simulink model "seminar3_1"  (R2019b)
settings: Solver=VariableStepAuto  StartTime=0.0  StopTime=0.1  RelTol=1e-3  EnableMultiTasking=on
model workspace (MAT data in the model file):
  thit = 150
values from neighbouring files (symbols this model uses):
  fai = i*10    [Untitled.m]
libraries: powerlib x16, powerlib_meascontrol x7
settings Model: Creator=Double Rui  LastModifiedBy=96547
settings DataIOCC: ReturnWorkspaceOutputs=off
settings OptimizationCC: LifeSpan=inf
settings DebuggingCC: SFUnexpectedBacktrackingDiag=warning  SFNoUnconditionalDefaultTransitionDiag=warning  ArithmeticOperatorsInVariantConditions=warning
settings SFSimCC: SimUseLocalCustomCode=off  CustomCodeUndefinedFunction=UseInterfaceOnly
settings RTWCC: RTWUseLocalCustomCode=off
settings CodeAppCC: StateflowObjectComments=on
settings GRTTargetCC: TargetLangStandard=C89/C90 (ANSI)  GeneratePreprocessorConditionals=Disable all
settings ConfigComp: CovMetricSettings=dw  CovHtmlReporting=on  CovSaveCumulativeToWorkspaceVar=on  CovSaveSingleToWorkspaceVar=on  CovExternalEMLEnable=off
settings SimscapeCC: SimscapeNormalizeSystem=off

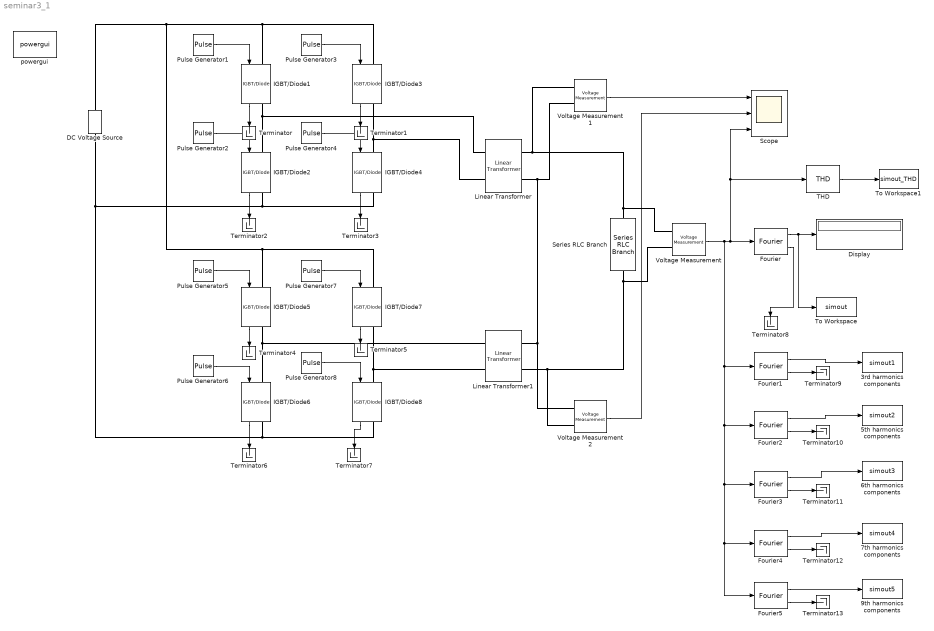
== system seminar3_1 ==
  3rd harmonics components : ToWorkspace  VariableName=simout1  SaveFormat=Timeseries  SampleTime=-1
  5th harmonics components : ToWorkspace  VariableName=simout2  SaveFormat=Timeseries  SampleTime=-1
  6th harmonics components : ToWorkspace  VariableName=simout3  SaveFormat=Timeseries  SampleTime=-1
  7th harmonics components : ToWorkspace  VariableName=simout4  SaveFormat=Timeseries  SampleTime=-1
  9th harmonics components : ToWorkspace  VariableName=simout5  SaveFormat=Timeseries  SampleTime=-1
  DC Voltage Source : powerlib/Electrical Sources/DC Voltage Source  Amplitude=400  Measurements=None
      settings: SourceProductName=Simscape Electrical
  Display : Display
  Fourier : powerlib_meascontrol/Measurements/Fourier  Freq=50  n=1  InInit=[0, 0]  Ts=0
      settings: SourceProductName=Simscape Electrical
  Fourier1 : powerlib_meascontrol/Measurements/Fourier  Freq=50  n=3  InInit=[0, 0]  Ts=0
      settings: SourceProductName=Simscape Electrical
  Fourier2 : powerlib_meascontrol/Measurements/Fourier  Freq=50  n=5  InInit=[0, 0]  Ts=0
      settings: SourceProductName=Simscape Electrical
  Fourier3 : powerlib_meascontrol/Measurements/Fourier  Freq=50  n=6  InInit=[0, 0]  Ts=0
      settings: SourceProductName=Simscape Electrical
  Fourier4 : powerlib_meascontrol/Measurements/Fourier  Freq=50  n=7  InInit=[0, 0]  Ts=0
      settings: SourceProductName=Simscape Electrical
  Fourier5 : powerlib_meascontrol/Measurements/Fourier  Freq=50  n=9  InInit=[0, 0]  Ts=0
      settings: SourceProductName=Simscape Electrical
  IGBT/Diode{1..8} (8 alike) : powerlib/Power Electronics/IGBT//Diode  Ron=1e-3  Rs=1e5  Cs=inf  Measurements=on
      settings: SourceProductName=Simscape Electrical
  Linear Transformer : powerlib/Elements/Linear Transformer  UNITS=pu  NominalPower=[ 250e6 50 ]  winding1="[ 735e3  0  0  ]"  winding2="[ 735e3  0  0 ]"  ThreeWindings=off  winding3=[ 315e3 0.002 0.08 ]  RmLm=[ 500 500 ]  Measurements=None  DataType=off
      settings: SourceProductName=Simscape Electrical
  Linear Transformer1 : powerlib/Elements/Linear Transformer  UNITS=pu  NominalPower=[ 250e6 50 ]  winding1="[ 735e3  0  0 ]"  winding2="[ 735e3  0  0 ]"  ThreeWindings=off  winding3=[ 315e3 0.002 0.08 ]  RmLm=[ 500 500 ]  Measurements=None  DataType=off
      settings: SourceProductName=Simscape Electrical
  Pulse Generator1 : DiscretePulseGenerator  PulseType=Time based  Period=0.02  PulseWidth=50  PhaseDelay=0.02/360*0
  Pulse Generator2 : DiscretePulseGenerator  PulseType=Time based  Period=0.02  PulseWidth=50  PhaseDelay=0.02/360*180
  Pulse Generator3 : DiscretePulseGenerator  PulseType=Time based  Period=0.02  PulseWidth=50  PhaseDelay=0.02/360*60
  Pulse Generator4 : DiscretePulseGenerator  PulseType=Time based  Period=0.02  PulseWidth=50  PhaseDelay=0.02/360*(180+60)
  Pulse Generator5 : DiscretePulseGenerator  PulseType=Time based  Period=0.02  PulseWidth=50  PhaseDelay=0.02/360*(0+fai)
  Pulse Generator6 : DiscretePulseGenerator  PulseType=Time based  Period=0.02  PulseWidth=50  PhaseDelay=0.02/360*(180+fai)
  Pulse Generator7 : DiscretePulseGenerator  PulseType=Time based  Period=0.02  PulseWidth=50  PhaseDelay=0.02/360*(60+fai)
  Pulse Generator8 : DiscretePulseGenerator  PulseType=Time based  Period=0.02  PulseWidth=50  PhaseDelay=0.02/360*(180+60+fai)
  Scope : Scope  NumInputPorts=3
  Series RLC Branch : powerlib/Elements/Series RLC Branch  LConnTagsString=__new0  RConnTagsString=__new0  BranchType=R  Resistance=8  Inductance=1e-3  SetiL0=off  InitialCurrent=0  Capacitance=1e-6  Setx0=off  InitialVoltage=0  Measurements=None
      settings: SourceProductName=Simscape Electrical
  THD : powerlib_meascontrol/Measurements/THD  Freq=60  Ts=0
      settings: SourceProductName=Simscape Electrical
  Terminator{,1..13} (14 alike) : Terminator
  To Workspace : ToWorkspace  VariableName=simout  SaveFormat=Timeseries  SampleTime=-1
  To Workspace1 : ToWorkspace  VariableName=simout_THD  SaveFormat=Timeseries  SampleTime=-1
  Voltage Measurement : powerlib/Measurements/Voltage Measurement  PhasorSimulation=off  OutputType=Complex  PSBequivalent=0
      settings: SourceProductName=Simscape Electrical
  Voltage Measurement1 : powerlib/Measurements/Voltage Measurement  PhasorSimulation=off  OutputType=Complex  PSBequivalent=0
      settings: SourceProductName=Simscape Electrical
  Voltage Measurement2 : powerlib/Measurements/Voltage Measurement  PhasorSimulation=off  OutputType=Complex  PSBequivalent=0
      settings: SourceProductName=Simscape Electrical
  powergui : powerlib/powergui  Priority=1  SimulationMode=Continuous  SampleTime=50e-6  frequency=60  Iterations=50  frequencyindice=0  Pbase=100e6  ErrMax=1e-4  UnitsV=kV  UnitsW=MW  buscounter=0  FunctionMessages=off  echomessages=off  EnableUseOfTLC=off  CurrentSourceSwitches=on  DisableSnubberDevices=off  DisableRonSwitches=off  DisableVfSwitches=off  DisplayEquations=off  AutomaticDiscreteSolvers=off  SolverType=Tustin/Backward Euler (TBE)  Interpol=off  ExternalGateDelay=off  methode=off  Ts=10  x0status=blocks  SPID=off  SwTol=0  HookPort=off  NonlinearTolerance=1e-4  nMaxIteration=100  ContinueOnMaxIteration=off  RestoreLinks=warning  ResistiveCurrentMeasurement=off  Frange=[0:2:500]  Ylog=off  Xlog=on  ShowGrid=off  save=off  variable=ZData  structure=ScopeData  ZoomFFT=off  StartTime=0.05  cycles=2  DisplayStyle=2  fundamental=50  FreqAxis=off  MaxFrequency=1000  frequencyindicesteady=1  RmsSteady=1  display=off
      settings: SourceProductName=Simscape Electrical
  wires:
  Pulse Generator1/1 -> IGBT/Diode1/1
  Pulse Generator3/1 -> IGBT/Diode3/1
  Pulse Generator2/1 -> IGBT/Diode2/1
  Pulse Generator4/1 -> IGBT/Diode4/1
  Pulse Generator5/1 -> IGBT/Diode5/1
  Pulse Generator7/1 -> IGBT/Diode7/1
  Pulse Generator6/1 -> IGBT/Diode6/1
  Pulse Generator8/1 -> IGBT/Diode8/1
  Voltage Measurement1/1 -> Scope/1
  Voltage Measurement2/1 -> Scope/2
  Voltage Measurement/1 -> THD/1, Scope/3, Fourier/1, Fourier3/1, Fourier4/1, Fourier5/1, Fourier2/1, Fourier1/1
  Fourier/1 -> To Workspace/1, Display/1
  IGBT/Diode1/1 -> Terminator/1
  IGBT/Diode3/1 -> Terminator1/1
  IGBT/Diode2/1 -> Terminator2/1
  IGBT/Diode4/1 -> Terminator3/1
  IGBT/Diode5/1 -> Terminator4/1
  IGBT/Diode7/1 -> Terminator5/1
  IGBT/Diode6/1 -> Terminator6/1
  IGBT/Diode8/1 -> Terminator7/1
  Fourier/2 -> Terminator8/1
  THD/1 -> To Workspace1/1
  Fourier1/2 -> Terminator9/1
  Fourier2/2 -> Terminator10/1
  Fourier3/2 -> Terminator11/1
  Fourier4/2 -> Terminator12/1
  Fourier5/2 -> Terminator13/1
  Fourier1/1 -> 3rd harmonics components/1
  Fourier2/1 -> 5th harmonics components/1
  Fourier3/1 -> 6th harmonics components/1
  Fourier4/1 -> 7th harmonics components/1
  Fourier5/1 -> 9th harmonics components/1
  connections:
  IGBT/Diode1/RConn1 -- Linear Transformer/LConn1 -- IGBT/Diode2/LConn1
  IGBT/Diode3/RConn1 -- Linear Transformer/LConn2 -- IGBT/Diode4/LConn1
  IGBT/Diode1/LConn1 -- IGBT/Diode7/LConn1 -- IGBT/Diode5/LConn1 -- DC Voltage Source/RConn1 -- IGBT/Diode3/LConn1
  IGBT/Diode2/RConn1 -- IGBT/Diode6/RConn1 -- IGBT/Diode8/RConn1 -- DC Voltage Source/LConn1 -- IGBT/Diode4/RConn1
  IGBT/Diode5/RConn1 -- IGBT/Diode6/LConn1 -- Linear Transformer1/LConn1
  IGBT/Diode7/RConn1 -- Linear Transformer1/LConn2 -- IGBT/Diode8/LConn1
  Linear Transformer/RConn2 -- Voltage Measurement2/LConn1 -- Linear Transformer1/RConn1 -- Voltage Measurement1/LConn2
  Linear Transformer/RConn1 -- Voltage Measurement1/LConn1 -- Voltage Measurement/LConn1 -- Series RLC Branch/LConn1
  Linear Transformer1/RConn2 -- Voltage Measurement2/LConn2 -- Voltage Measurement/LConn2 -- Series RLC Branch/RConn1
